simulink model "s0218d"  (Simulink 6.0)
settings: Solver=ode45  SolverMode=SingleTasking  StartTime=0.0  StopTime=5  MaxStep=.1  RelTol=1e-3  AbsTol=1e-6
values from neighbouring files (symbols this model uses):
  Domdach = DomdachVec(i)    [m0218e.m]
  l = l*1e-2    (= 0.1)    [m0212d.m]    (also in m0218a.m; m0218e.m; m0251.m = 0.2; m0252.m = 0.2)
  phi0 = (pi/180)*phi0Grad    (= 0.785398163397)    [m0218a.m]    (also in m0218e.m)
  rP = rP*1e-2    (= 0.01)    [m0212d.m]    (also in m0218a.m; m0218e.m)
  tsprung = .5    (= 0.5)    [m0218e.m]
settings Model: LastModifiedBy=Froriep
settings DataIOCC: LimitDataPoints=off  SaveOutput=off  TimeSaveName=t
settings OptimizationCC: BooleanDataType=off
settings DebuggingCC: SolverPrmCheckMsg=none
settings HardwareCC: TargetUnknown=on
settings GRTTargetCC: ModelReferenceCompliant=off  MatFileLogging=off

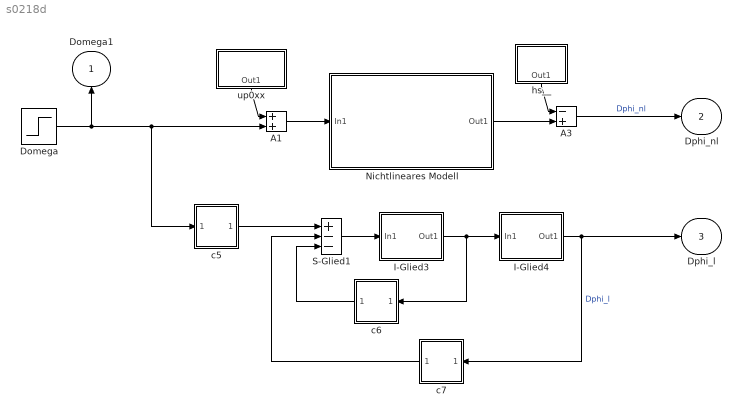
== system s0218d ==
  A1 : Sum  SaturateOnIntegerOverflow=on  InputSameDT=on
  A3 : Sum  Inputs=-+  SaturateOnIntegerOverflow=on  InputSameDT=on
  Domega : Step  Time=tsprung  After=Domdach  SampleTime=0
  I-Glied3 : Subsystem  mask(I-Glied){@1=0}
      mask prompts: @1 "Anfangswert"
      mask help: I-Glied
      mask init:
      | x0=@1;
      mask Display: disp('I-Glied')
  I-Glied4 : Subsystem  mask(I-Glied){@1=0}
      mask prompts: @1 "Anfangswert"
      mask help: I-Glied
      mask init:
      | x0=@1;
      mask Display: disp('I-Glied')
  Nichtlineares Modell : Subsystem
      mask Display: disp('Nichtlineares\n Fliehkraftpendel-\nmodell')
  S-Glied1 : Sum  Inputs=+--  SaturateOnIntegerOverflow=on  InputSameDT=on
  c5 : Subsystem  mask(P-Glied){@1=b0}
      mask prompts: @1 "Beiwert"
      mask help: P-Glied
      mask init:
      | Kp=@1;
      mask Display: disp('b0')
  c6 : Subsystem  Orientation=left  mask(P-Glied){@1=a1}
      mask prompts: @1 "Beiwert"
      mask help: P-Glied
      mask init:
      | Kp=@1;
      mask Display: disp('a1')
  c7 : Subsystem  Orientation=left  mask(P-Glied){@1=a0}
      mask prompts: @1 "Beiwert"
      mask help: P-Glied
      mask init:
      | Kp=@1;
      mask Display: disp('a0')
  hs__ : Subsystem  Orientation=down  mask(Konstante){@1=phi0}
      mask prompts: @1 "Wert"
      mask help: Konstante
      mask init:
      | Konst=@1;
      mask Display: disp('phi0')
  up0xx : Subsystem  Orientation=down  mask(Konstante){@1=omega0}
      mask prompts: @1 "Wert"
      mask help: Konstante
      mask init:
      | Konst=@1;
      mask Display: disp('omega0')
  Domega1 : Outport  Orientation=up
  Dphi_nl : Outport  Port=2
  Dphi_l : Outport  Port=3
  wires:
  up0xx/1(Out1) -> A1/1
  hs__/1(Out1) -> A3/1
  A1/1 -> Nichtlineares Modell/1(In1)
  Domega/1 -> Domega1/1, A1/2, c5/1(In1)
  A3/1 -> Dphi_nl/1  "Dphi_nl"
  c6/1(Out1) -> S-Glied1/3
  I-Glied3/1(Out1) -> I-Glied4/1(In1), c6/1(In1)
  S-Glied1/1 -> I-Glied3/1(In1)
  c5/1(Out1) -> S-Glied1/1
  c7/1(Out1) -> S-Glied1/2
  I-Glied4/1(Out1) -> c7/1(In1), Dphi_l/1  "Dphi_l"
  Nichtlineares Modell/1(Out1) -> A3/2

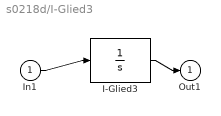
== system s0218d/I-Glied3 ==
  In1 : Inport  Port=1  LatchInput=off
  I-Glied3 : Integrator  InitialCondition=x0
  Out1 : Outport
  wires:
  In1/1 -> I-Glied3/1
  I-Glied3/1 -> Out1/1

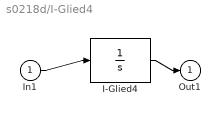
== system s0218d/I-Glied4 ==
  In1 : Inport  Port=1  LatchInput=off
  I-Glied4 : Integrator  InitialCondition=x0
  Out1 : Outport
  wires:
  In1/1 -> I-Glied4/1
  I-Glied4/1 -> Out1/1

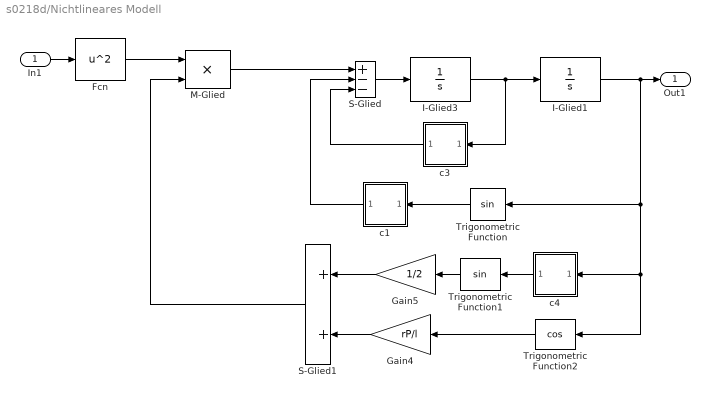
== system s0218d/Nichtlineares Modell ==
  In1 : Inport  Port=1  LatchInput=off
  Fcn : Fcn  Expr=u^2
  Gain4 : Gain  Orientation=left  Gain=rP/l
  Gain5 : Gain  Orientation=left  Gain=1/2
  I-Glied1 : Integrator  InitialCondition=phi0
  I-Glied3 : Integrator
  M-Glied : Product  SaturateOnIntegerOverflow=on  RndMeth=Zero  InputSameDT=on
  S-Glied : Sum  Inputs=+--  SaturateOnIntegerOverflow=on  InputSameDT=on
  S-Glied1 : Sum  Orientation=left  SaturateOnIntegerOverflow=on  InputSameDT=on
  Trigonometric Function : Trigonometry  Orientation=left
  Trigonometric Function1 : Trigonometry  Orientation=left
  Trigonometric Function2 : Trigonometry  Orientation=left  Operator=cos
  c1 : Subsystem  Orientation=left  mask(P-Glied){@1=c2}
      mask prompts: @1 "Beiwert"
      mask help: P-Glied
      mask init:
      | Kp=@1;
      mask Display: disp('c2')
  c3 : Subsystem  Orientation=left  mask(P-Glied){@1=c1}
      mask prompts: @1 "Beiwert"
      mask help: P-Glied
      mask init:
      | Kp=@1;
      mask Display: disp('c1')
  c4 : Subsystem  Orientation=left  mask(P-Glied){@1=2}
      mask prompts: @1 "Beiwert"
      mask help: P-Glied
      mask init:
      | Kp=@1;
      mask Display: disp('2')
  Out1 : Outport
  wires:
  S-Glied/1 -> I-Glied3/1
  M-Glied/1 -> S-Glied/1
  Fcn/1 -> M-Glied/1
  I-Glied3/1 -> c3/1(In1), I-Glied1/1
  c3/1(Out1) -> S-Glied/3
  c1/1(Out1) -> S-Glied/2
  Trigonometric Function/1 -> c1/1(In1)
  c4/1(Out1) -> Trigonometric Function1/1
  I-Glied1/1 -> Trigonometric Function/1, c4/1(In1), Trigonometric Function2/1, Out1/1
  In1/1 -> Fcn/1
  Gain4/1 -> S-Glied1/2
  Gain5/1 -> S-Glied1/1
  Trigonometric Function1/1 -> Gain5/1
  Trigonometric Function2/1 -> Gain4/1
  S-Glied1/1 -> M-Glied/2

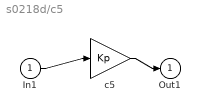
== system s0218d/c5 ==
  In1 : Inport  Port=1  LatchInput=off
  c5 : Gain  Gain=Kp  SaturateOnIntegerOverflow=on
  Out1 : Outport
  wires:
  In1/1 -> c5/1
  c5/1 -> Out1/1

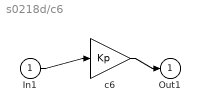
== system s0218d/c6 ==
  In1 : Inport  Port=1  LatchInput=off
  c6 : Gain  Gain=Kp  SaturateOnIntegerOverflow=on
  Out1 : Outport
  wires:
  In1/1 -> c6/1
  c6/1 -> Out1/1

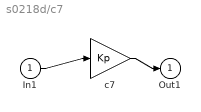
== system s0218d/c7 ==
  In1 : Inport  Port=1  LatchInput=off
  c7 : Gain  Gain=Kp  SaturateOnIntegerOverflow=on
  Out1 : Outport
  wires:
  In1/1 -> c7/1
  c7/1 -> Out1/1

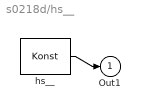
== system s0218d/hs__ ==
  hs__ : Constant  Value=Konst
  Out1 : Outport
  wires:
  hs__/1 -> Out1/1

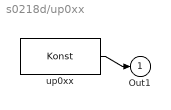
== system s0218d/up0xx ==
  up0xx : Constant  Value=Konst
  Out1 : Outport
  wires:
  up0xx/1 -> Out1/1

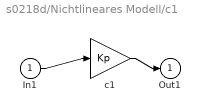
== system s0218d/Nichtlineares Modell/c1 ==
  In1 : Inport  Port=1  LatchInput=off
  c1 : Gain  Gain=Kp  SaturateOnIntegerOverflow=on
  Out1 : Outport
  wires:
  In1/1 -> c1/1
  c1/1 -> Out1/1

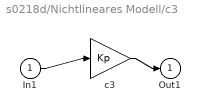
== system s0218d/Nichtlineares Modell/c3 ==
  In1 : Inport  Port=1  LatchInput=off
  c3 : Gain  Gain=Kp  SaturateOnIntegerOverflow=on
  Out1 : Outport
  wires:
  In1/1 -> c3/1
  c3/1 -> Out1/1

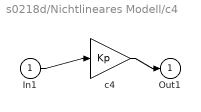
== system s0218d/Nichtlineares Modell/c4 ==
  In1 : Inport  Port=1  LatchInput=off
  c4 : Gain  Gain=Kp  SaturateOnIntegerOverflow=on
  Out1 : Outport
  wires:
  In1/1 -> c4/1
  c4/1 -> Out1/1
